simulink model "sf_variable_size_data"  (R2017b)
settings: Solver=FixedStepDiscrete  StartTime=0.0  StopTime=5.0  RelTol=1e-3  EnableMultiTasking=on
settings Model: Creator=The MathWorks, Inc.  LastModifiedBy=The MathWorks, Inc.
settings DataIOCC: LimitDataPoints=on  SaveFormat=Array
settings OptimizationCC: ExpressionDepthLimit=2147483647  LifeSpan=inf
settings DebuggingCC: UnderspecifiedInitializationDetection=Classic  MergeDetectMultiDrivingBlocksExec=none  FcnCallInpInsideContextMsg=warning  StateNameClashWarn=warning  StrictBusMsg=Warning  SFUnexpectedBacktrackingDiag=warning  SFNoUnconditionalDefaultTransitionDiag=warning  SFExecutionAtInitializationDiag=none
settings HardwareCC: ProdBitPerPointer=32  ProdBitPerSizeT=32  ProdBitPerPtrDiffT=32  ProdLargestAtomicFloat=None  ProdIntDivRoundTo=Undefined  ProdEndianess=Unspecified  ProdWordSize=32  ProdHWDeviceType=32-bit Generic
settings ModelReferenceCC: PropagateSignalLabelsOutOfModel=off
settings SFSimCC: SFSimEcho=off  SimParseCustomCode=off
settings CodeAppCC: StateflowObjectComments=on
settings GRTTargetCC: TargetLangStandard=C89/C90 (ANSI)  GeneratePreprocessorConditionals=Disable all  CombineOutputUpdateFcns=off  GRTInterface=on
settings ConfigComp: CovMetricSettings=dw  CovHtmlReporting=on  CovSaveCumulativeToWorkspaceVar=on  CovSaveSingleToWorkspaceVar=on  CovExternalEMLEnable=off  CovSFcnEnable=off

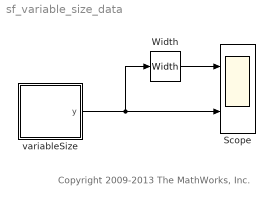
== system sf_variable_size_data ==
  note: Copyright 2009-2013 The MathWorks, Inc.
  Scope : Scope  NumInputPorts=2
  Width : Width
  variableSize : Stateflow chart  TreatAsAtomicUnit=on
  wires:
  Width/1 -> Scope/1
  variableSize/1(y) -> Scope/2, Width/1

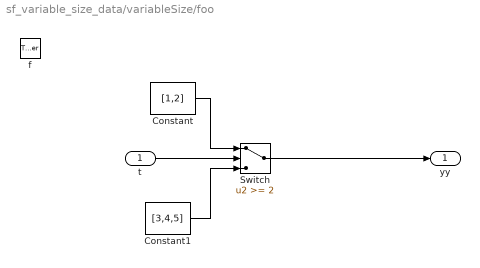
== system sf_variable_size_data/variableSize/foo ==
  t : Inport
  f : TriggerPort  TriggerType=function-call  VariantControl=(inherit)
      settings: CopyFcn=Stateflow.SLINSF.SimulinkMan.removeBlockPreDeleteFcn  PreDeleteFcn=Stateflow.SLINSF.SimulinkMan.unsafePredeleteFcn
  Constant : Constant  Value=[1,2]
  Constant1 : Constant  Value=[3,4,5]
  Switch : Switch  Threshold=2  AllowDiffInputSizes=on
  yy : Outport
  wires:
  Constant/1 -> Switch/1
  t/1 -> Switch/2
  Constant1/1 -> Switch/3
  Switch/1 -> yy/1

== stateflow chart sf_variable_size_data/variableSize ==
  settings: updateMethod=DISCRETE  sampleTime=.1
  state yy = foo(t) [function]
  (default) -> (junction 2) : {y = foo(t);}
  data: yy function_output; t function_input; y output double size=3
